simulink model "Week2_problem2"  (R2020b)
settings: Solver=VariableStepAuto  StartTime=0.0  StopTime=10.0  RelTol=1e-3
undefined symbols (not defined in the file): be, bv, Ie, Iv, muk, mus, R
settings Model: DataDictionary=datadictionary.sldd  Creator=Gauri  LastModifiedBy=mluser

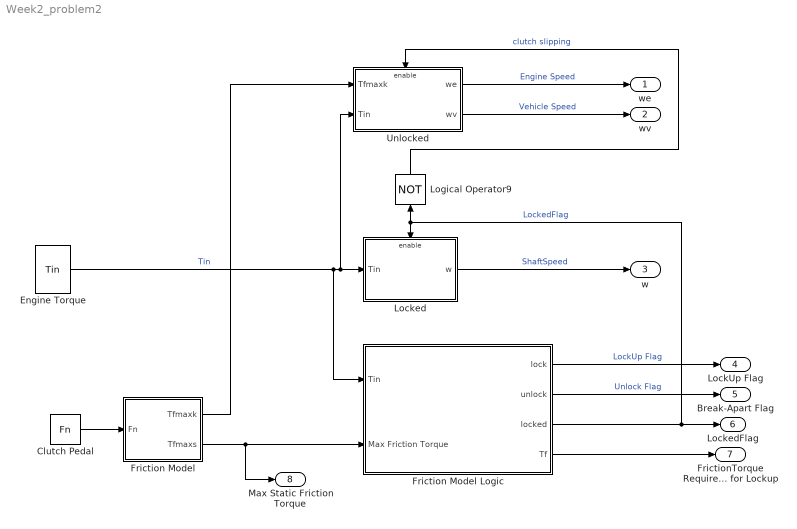
== system Week2_problem2 ==
  Clutch Pedal : FromWorkspace  VariableName=Fn  ZeroCross=off
  Engine Torque : FromWorkspace  VariableName=Tin  ZeroCross=off
  Friction Model : Subsystem
  Friction Model Logic : Subsystem
  Locked : Subsystem
  Logical Operator9 : Logic  Operator=NOT  Inputs=1  IconShape=distinctive  OutDataTypeStr=boolean
  Unlocked : Subsystem
  we : Outport  InitialOutput=0  VectorParamsAs1DForOutWhenUnconnected=off
  wv : Outport  Port=2  InitialOutput=0  VectorParamsAs1DForOutWhenUnconnected=off
  w : Outport  Port=3  InitialOutput=0  VectorParamsAs1DForOutWhenUnconnected=off
  LockUp Flag : Outport  Port=4  InitialOutput=0  VectorParamsAs1DForOutWhenUnconnected=off
  Break-Apart Flag : Outport  Port=5  InitialOutput=0  VectorParamsAs1DForOutWhenUnconnected=off
  LockedFlag : Outport  Port=6  InitialOutput=0  VectorParamsAs1DForOutWhenUnconnected=off
  FrictionTorque Required for Lockup : Outport  Port=7  InitialOutput=0  VectorParamsAs1DForOutWhenUnconnected=off
  Max Static Friction Torque : Outport  Port=8  InitialOutput=0  VectorParamsAs1DForOutWhenUnconnected=off
  wires:
  Clutch Pedal/1 -> Friction Model/1(Fn)
  Logical Operator9/1 -> Unlocked/Enable  "clutch slipping"
  Friction Model Logic/3(locked) -> Logical Operator9/1, Locked/Enable, LockedFlag/1  "LockedFlag"
  Engine Torque/1 -> Friction Model Logic/1(Tin), Unlocked/2(Tin), Locked/1(Tin)  "Tin"
  Locked/1(w) -> w/1  "ShaftSpeed"
  Friction Model Logic/1(lock) -> LockUp Flag/1  "LockUp Flag"
  Friction Model Logic/2(unlock) -> Break-Apart Flag/1  "Unlock Flag"
  Unlocked/2(wv) -> wv/1  "Vehicle Speed"
  Friction Model Logic/4(Tf) -> FrictionTorque Required for Lockup/1
  Friction Model/2(Tfmaxs) -> Max Static Friction Torque/1, Friction Model Logic/2(Max Friction Torque)
  Friction Model/1(Tfmaxk) -> Unlocked/1(Tfmaxk)
  Unlocked/1(we) -> we/1  "Engine Speed"

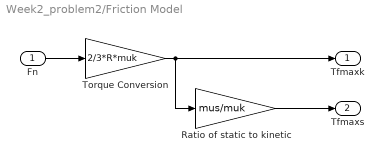
== system Week2_problem2/Friction Model ==
  Fn : Inport
  Ratio of static to kinetic : Gain  Gain=mus/muk  SaturateOnIntegerOverflow=on  OutDataTypeStr=Inherit: Same as input  ParamDataTypeStr=Inherit: Same as input
  Torque Conversion : Gain  Gain=2/3*R*muk  SaturateOnIntegerOverflow=on  OutDataTypeStr=Inherit: Same as input  ParamDataTypeStr=Inherit: Same as input
  Tfmaxk : Outport  InitialOutput=0  VectorParamsAs1DForOutWhenUnconnected=off
  Tfmaxs : Outport  Port=2  InitialOutput=0  VectorParamsAs1DForOutWhenUnconnected=off
  wires:
  Torque Conversion/1 -> Tfmaxk/1, Ratio of static to kinetic/1
  Ratio of static to kinetic/1 -> Tfmaxs/1
  Fn/1 -> Torque Conversion/1

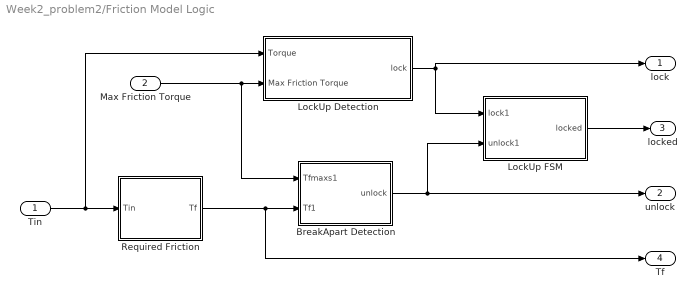
== system Week2_problem2/Friction Model Logic ==
  Tin : Inport
  Max Friction Torque : Inport  Port=2
  BreakApart Detection : Subsystem
  LockUp Detection : Subsystem
  LockUp FSM : Subsystem
  Required Friction : Subsystem
  lock : Outport  InitialOutput=0  VectorParamsAs1DForOutWhenUnconnected=off
  unlock : Outport  Port=2  InitialOutput=0  VectorParamsAs1DForOutWhenUnconnected=off
  locked : Outport  Port=3  InitialOutput=0  VectorParamsAs1DForOutWhenUnconnected=off
  Tf : Outport  Port=4  InitialOutput=0  VectorParamsAs1DForOutWhenUnconnected=off
  wires:
  Max Friction Torque/1 -> BreakApart Detection/1(Tfmaxs1), LockUp Detection/2(Max Friction Torque)
  Required Friction/1(Tf) -> Tf/1, BreakApart Detection/2(Tf1)
  LockUp FSM/1(locked) -> locked/1
  Tin/1 -> LockUp Detection/1(Torque), Required Friction/1(Tin)
  LockUp Detection/1(lock) -> lock/1, LockUp FSM/1(lock1)
  BreakApart Detection/1(unlock) -> unlock/1, LockUp FSM/2(unlock1)

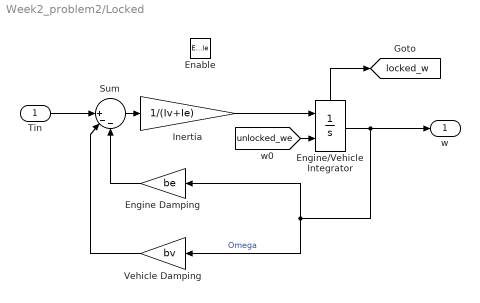
== system Week2_problem2/Locked ==
  Tin : Inport
  Enable : EnablePort  StatesWhenEnabling=reset
  Engine Damping : Gain  Gain=be  SaturateOnIntegerOverflow=on  OutDataTypeStr=Inherit: Same as input  ParamDataTypeStr=Inherit: Same as input
  Engine/Vehicle Integrator : Integrator  InitialConditionSource=external  ShowStatePort=on
  Inertia : Gain  Gain=1/(Iv+Ie)  SaturateOnIntegerOverflow=on  OutDataTypeStr=Inherit: Same as input  ParamDataTypeStr=Inherit: Same as input
  Sum : Sum  Inputs=||+--  InputSameDT=on  SaturateOnIntegerOverflow=on  OutDataTypeStr=Inherit: Same as first input
  Vehicle Damping : Gain  Gain=bv  SaturateOnIntegerOverflow=on  OutDataTypeStr=Inherit: Same as input  ParamDataTypeStr=Inherit: Same as input
  w : Outport  InitialOutput=0  VectorParamsAs1DForOutWhenUnconnected=off
  tag scope: locked_w=global
  wires:
  Engine/Vehicle Integrator/State -> [locked_w]
  Inertia/1 -> Engine/Vehicle Integrator/1
  Engine Damping/1 -> Sum/3
  Engine/Vehicle Integrator/1 -> w/1, Engine Damping/1, Vehicle Damping/1  "Omega"
  [unlocked_we] -> Engine/Vehicle Integrator/2
  Sum/1 -> Inertia/1
  Vehicle Damping/1 -> Sum/2
  Tin/1 -> Sum/1

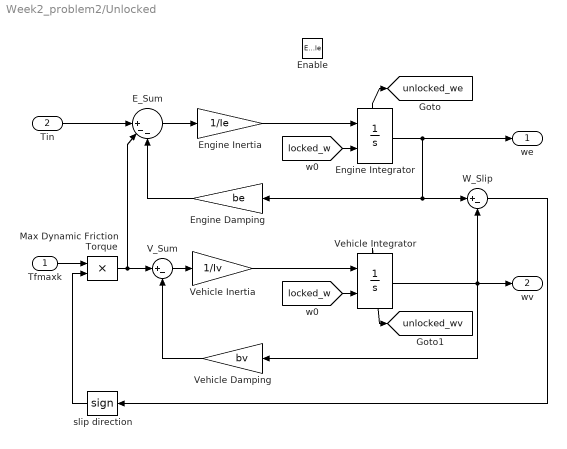
== system Week2_problem2/Unlocked ==
  Tfmaxk : Inport
  Tin : Inport  Port=2
  Enable : EnablePort  StatesWhenEnabling=reset
  E_Sum : Sum  Inputs=||+--  InputSameDT=on  SaturateOnIntegerOverflow=on  OutDataTypeStr=Inherit: Same as first input
  Engine Damping : Gain  Gain=be  SaturateOnIntegerOverflow=on  OutDataTypeStr=Inherit: Same as input  ParamDataTypeStr=Inherit: Same as input
  Engine Inertia : Gain  Gain=1/Ie  SaturateOnIntegerOverflow=on  OutDataTypeStr=Inherit: Same as input  ParamDataTypeStr=Inherit: Same as input
  Engine Integrator : Integrator  InitialConditionSource=external  ShowStatePort=on
  Max Dynamic Friction Torque : Product  InputSameDT=on  RndMeth=Zero  SaturateOnIntegerOverflow=on  OutDataTypeStr=Inherit: Same as first input
  V_Sum : Sum  Inputs=|+-  InputSameDT=on  SaturateOnIntegerOverflow=on  OutDataTypeStr=Inherit: Same as first input
  Vehicle Damping : Gain  Gain=bv  SaturateOnIntegerOverflow=on  OutDataTypeStr=Inherit: Same as input  ParamDataTypeStr=Inherit: Same as input
  Vehicle Inertia : Gain  Gain=1/Iv  SaturateOnIntegerOverflow=on  OutDataTypeStr=Inherit: Same as input  ParamDataTypeStr=Inherit: Same as input
  Vehicle Integrator : Integrator  InitialConditionSource=external  ShowStatePort=on
  W_Slip : Sum  Inputs=|+-  InputSameDT=on  SaturateOnIntegerOverflow=on  OutDataTypeStr=Inherit: Same as first input
  slip direction : Signum
  we : Outport  InitialOutput=0  VectorParamsAs1DForOutWhenUnconnected=off
  wv : Outport  Port=2  InitialOutput=0  VectorParamsAs1DForOutWhenUnconnected=off
  tag scope: unlocked_we=global, unlocked_wv=global
  wires:
  Vehicle Integrator/1 -> wv/1, W_Slip/2, Vehicle Damping/1
  slip direction/1 -> Max Dynamic Friction Torque/2
  E_Sum/1 -> Engine Inertia/1
  Vehicle Integrator/State -> [unlocked_wv]
  Vehicle Damping/1 -> V_Sum/2
  Max Dynamic Friction Torque/1 -> V_Sum/1, E_Sum/2
  V_Sum/1 -> Vehicle Inertia/1
  Vehicle Inertia/1 -> Vehicle Integrator/1
  [locked_w] -> Engine Integrator/2
  Tfmaxk/1 -> Max Dynamic Friction Torque/1
  Engine Damping/1 -> E_Sum/3
  Tin/1 -> E_Sum/1
  [locked_w] -> Vehicle Integrator/2
  Engine Integrator/State -> [unlocked_we]
  Engine Integrator/1 -> we/1, Engine Damping/1, W_Slip/1
  Engine Inertia/1 -> Engine Integrator/1
  W_Slip/1 -> slip direction/1

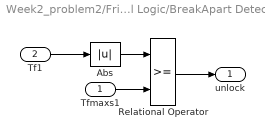
== system Week2_problem2/Friction Model Logic/BreakApart Detection ==
  Tfmaxs1 : Inport
  Tf1 : Inport  Port=2
  Abs : Abs  SaturateOnIntegerOverflow=on
  Relational Operator : RelationalOperator  OutDataTypeStr=boolean  RndMeth=Nearest  InputSameDT=on
  unlock : Outport  InitialOutput=0  VectorParamsAs1DForOutWhenUnconnected=off
  wires:
  Abs/1 -> Relational Operator/1
  Relational Operator/1 -> unlock/1
  Tfmaxs1/1 -> Relational Operator/2
  Tf1/1 -> Abs/1

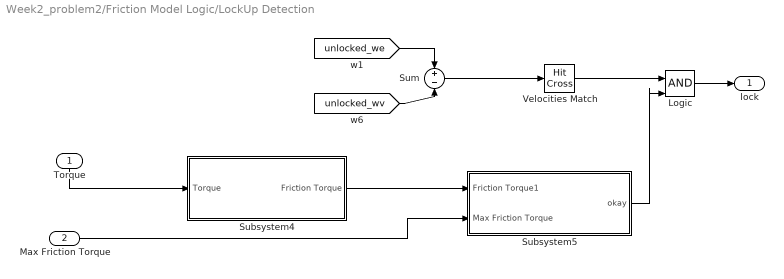
== system Week2_problem2/Friction Model Logic/LockUp Detection ==
  Torque : Inport
  Max Friction Torque : Inport  Port=2
  Logic : Logic  IconShape=distinctive  OutDataTypeStr=boolean
  Subsystem4 : Subsystem
  Subsystem5 : Subsystem
  Sum : Sum  Inputs=+-  InputSameDT=on  SaturateOnIntegerOverflow=on  OutDataTypeStr=Inherit: Same as first input
  Velocities Match : HitCross
  lock : Outport  InitialOutput=0  VectorParamsAs1DForOutWhenUnconnected=off
  wires:
  Velocities Match/1 -> Logic/1
  [unlocked_we] -> Sum/1
  [unlocked_wv] -> Sum/2
  Subsystem4/1(Friction Torque) -> Subsystem5/1(Friction Torque1)
  Sum/1 -> Velocities Match/1
  Logic/1 -> lock/1
  Torque/1 -> Subsystem4/1(Torque)
  Max Friction Torque/1 -> Subsystem5/2(Max Friction Torque)
  Subsystem5/1(okay) -> Logic/2

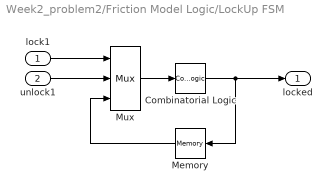
== system Week2_problem2/Friction Model Logic/LockUp FSM ==
  lock1 : Inport
  unlock1 : Inport  Port=2
  Combinatorial Logic : CombinatorialLogic  TruthTable=[0;1;0;0;1;1;1;0]
  Memory : Memory
  Mux : Mux  Inputs=3
  locked : Outport  InitialOutput=0  VectorParamsAs1DForOutWhenUnconnected=off
  wires:
  lock1/1 -> Mux/1
  Memory/1 -> Mux/3
  Mux/1 -> Combinatorial Logic/1
  Combinatorial Logic/1 -> locked/1, Memory/1
  unlock1/1 -> Mux/2

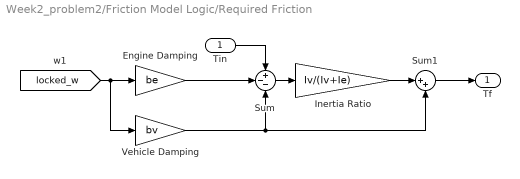
== system Week2_problem2/Friction Model Logic/Required Friction ==
  Tin : Inport
  Engine Damping : Gain  Gain=be  SaturateOnIntegerOverflow=on  OutDataTypeStr=Inherit: Same as input  ParamDataTypeStr=Inherit: Same as input
  Inertia Ratio : Gain  Gain=Iv/(Iv+Ie)  SaturateOnIntegerOverflow=on  OutDataTypeStr=Inherit: Same as input  ParamDataTypeStr=Inherit: Same as input
  Sum : Sum  Inputs=+--  InputSameDT=on  SaturateOnIntegerOverflow=on  OutDataTypeStr=Inherit: Same as first input
  Sum1 : Sum  Inputs=|++  InputSameDT=on  SaturateOnIntegerOverflow=on  OutDataTypeStr=Inherit: Same as first input
  Vehicle Damping : Gain  Gain=bv  SaturateOnIntegerOverflow=on  OutDataTypeStr=Inherit: Same as input  ParamDataTypeStr=Inherit: Same as input
  Tf : Outport  InitialOutput=0  VectorParamsAs1DForOutWhenUnconnected=off
  wires:
  Inertia Ratio/1 -> Sum1/1
  Tin/1 -> Sum/1
  Sum1/1 -> Tf/1
  Sum/1 -> Inertia Ratio/1
  Vehicle Damping/1 -> Sum/3, Sum1/2
  [locked_w] -> Vehicle Damping/1, Engine Damping/1
  Engine Damping/1 -> Sum/2

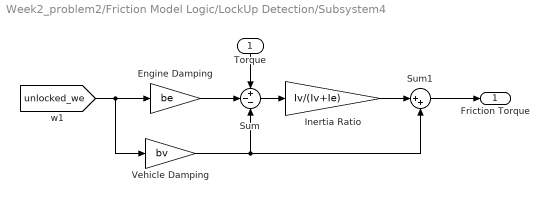
== system Week2_problem2/Friction Model Logic/LockUp Detection/Subsystem4 ==
  Torque : Inport
  Engine Damping : Gain  Gain=be  SaturateOnIntegerOverflow=on  OutDataTypeStr=Inherit: Same as input  ParamDataTypeStr=Inherit: Same as input
  Inertia Ratio : Gain  Gain=Iv/(Iv+Ie)  SaturateOnIntegerOverflow=on  OutDataTypeStr=Inherit: Same as input  ParamDataTypeStr=Inherit: Same as input
  Sum : Sum  Inputs=+--  InputSameDT=on  SaturateOnIntegerOverflow=on  OutDataTypeStr=Inherit: Same as first input
  Sum1 : Sum  Inputs=|++  InputSameDT=on  SaturateOnIntegerOverflow=on  OutDataTypeStr=Inherit: Same as first input
  Vehicle Damping : Gain  Gain=bv  SaturateOnIntegerOverflow=on  OutDataTypeStr=Inherit: Same as input  ParamDataTypeStr=Inherit: Same as input
  Friction Torque : Outport  InitialOutput=0  VectorParamsAs1DForOutWhenUnconnected=off
  wires:
  Vehicle Damping/1 -> Sum1/2, Sum/3
  Inertia Ratio/1 -> Sum1/1
  [unlocked_we] -> Engine Damping/1, Vehicle Damping/1
  Sum/1 -> Inertia Ratio/1
  Torque/1 -> Sum/1
  Sum1/1 -> Friction Torque/1
  Engine Damping/1 -> Sum/2

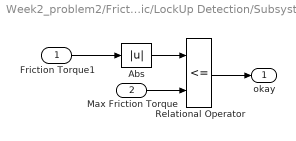
== system Week2_problem2/Friction Model Logic/LockUp Detection/Subsystem5 ==
  Friction Torque1 : Inport
  Max Friction Torque : Inport  Port=2
  Abs : Abs  SaturateOnIntegerOverflow=on
  Relational Operator : RelationalOperator  Operator=<=  OutDataTypeStr=boolean  RndMeth=Nearest  InputSameDT=on
  okay : Outport  InitialOutput=0  VectorParamsAs1DForOutWhenUnconnected=off
  wires:
  Relational Operator/1 -> okay/1
  Abs/1 -> Relational Operator/1
  Friction Torque1/1 -> Abs/1
  Max Friction Torque/1 -> Relational Operator/2
